simulink model "CrashAlgo_TestEnvironment_Cobi_v1"  (R2020b)
settings: Solver=FixedStepAuto  StartTime=0.0  StopTime=seconds(data.t(end))  FixedStep=0.01  RelTol=1e-3
values from neighbouring files (symbols this model uses):
  CrashClass = <binary blob, 4098 chars, not shown>    [CRCL_Dictionary.sldd]
undefined symbols (not defined in the file or in its folder): data
settings Model: SimulationMode=accelerator  Creator=snj7rt  LastModifiedBy=HNA3SI
settings DebuggingCC: ReadBeforeWriteMsg=DisableAll  WriteAfterWriteMsg=DisableAll  WriteAfterReadMsg=DisableAll  ParameterPrecisionLossMsg=none  ArithmeticOperatorsInVariantConditions=warning
settings ModelReferenceCC: UpdateModelReferenceTargets=IfOutOfDate
settings SFSimCC: SimUseLocalCustomCode=off  CustomCodeUndefinedFunction=UseInterfaceOnly
settings RTWCC: RTWUseLocalCustomCode=off
settings CodeAppCC: StateflowObjectComments=on

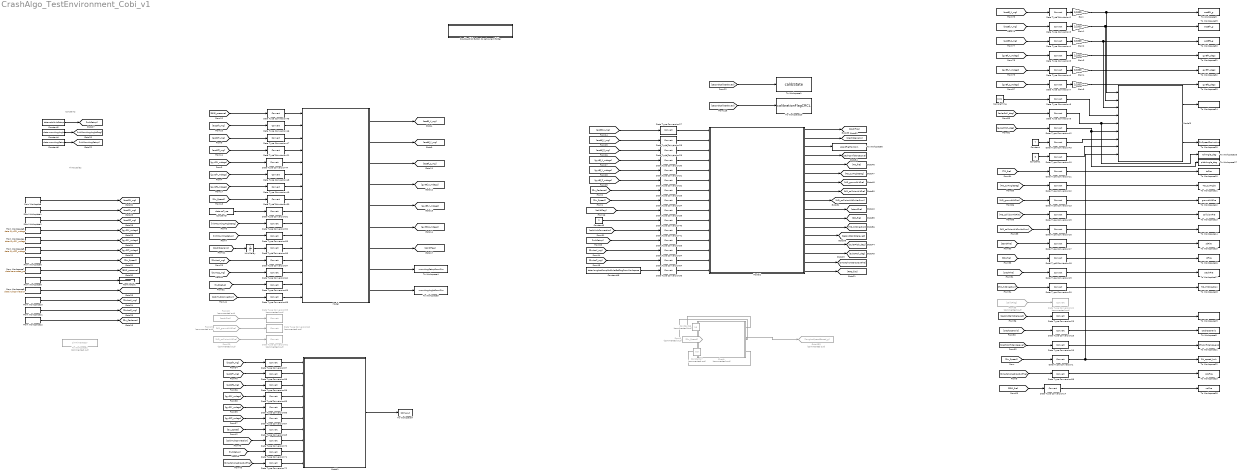
== system CrashAlgo_TestEnvironment_Cobi_v1 ==
  note: Time series
  note: Constants
  Chart1 : Stateflow chart  Commented=on  TreatAsAtomicUnit=on
  Constant : Constant  Value=7
  Constant1 : Constant  Value=5
  Constant2 : Constant  Value=data.cobiHubSetup
  Constant3 : Constant  Value=2
  Constant4 : Constant  Value=data.mountingAngle
  Constant46 : Constant  Commented=on  Value=15
  Constant47 : Constant  Commented=on  Value=0.5
  Constant48 : Constant  Value=data.longAccCompForEulerEstFlagFromWorkspace
  Constant5 : Constant  Value=data.osType
  Constant6 : Constant  Value=data.mountingSetup
  Data Type Conversion{1..20,23,25..26,42..43,58} (26 alike) : DataTypeConversion
  Data Type Conversion{21,27..41,44..57,62..72} (41 alike) : DataTypeConversion  RndMeth=Zero
  Data Type Conversion{22,59..61} (4 alike) : DataTypeConversion  Commented=on
  Double-Click Button to set current folder : Subsystem
      settings: OpenFcn=cd(fileparts(get_param(gcs,'filename')));
      mask Display: disp('\bf\fontsize{16}Double-Click to set current folder      ','texmode','on')
  From Workspace : FromWorkspace  VariableName=data.AccSfX_mg  SampleTime=0.01  Interpolate=off  ZeroCross=off  OutputAfterFinalValue=Setting to zero
  From Workspace1 : FromWorkspace  VariableName=data.AccSfY_mg  SampleTime=0.01  Interpolate=off  ZeroCross=off  OutputAfterFinalValue=Setting to zero
  From Workspace10 : FromWorkspace  VariableName=data.DuAccX_mg  SampleTime=0.01  Interpolate=off  ZeroCross=off  OutputAfterFinalValue=Setting to zero
  From Workspace11 : FromWorkspace  VariableName=data.DuAccZ_mg  SampleTime=0.01  Interpolate=off  ZeroCross=off  OutputAfterFinalValue=Setting to zero
  From Workspace12 : FromWorkspace  VariableName=data.cadence_rpm  SampleTime=0.01  Interpolate=off  ZeroCross=off  OutputAfterFinalValue=Setting to zero
  From Workspace2 : FromWorkspace  VariableName=data.AccSfZ_mg  SampleTime=0.01  Interpolate=off  ZeroCross=off  OutputAfterFinalValue=Setting to zero
  From Workspace3 : FromWorkspace  VariableName=data.GyrSfX_mdegs  SampleTime=0.01  Interpolate=off  ZeroCross=off  OutputAfterFinalValue=Setting to zero
  From Workspace4 : FromWorkspace  VariableName=data.GyrSfY_mdegs  SampleTime=0.01  Interpolate=off  ZeroCross=off  OutputAfterFinalValue=Setting to zero
  From Workspace5 : FromWorkspace  VariableName=data.GyrSfZ_mdegs  SampleTime=0.01  Interpolate=off  ZeroCross=off  OutputAfterFinalValue=Setting to zero
  From Workspace6 : FromWorkspace  VariableName=data.speed_kmh  SampleTime=0.01  Interpolate=off  ZeroCross=off  OutputAfterFinalValue=Setting to zero
  From Workspace7 : FromWorkspace  VariableName=data.barometer_pa  SampleTime=0.01  Interpolate=off  ZeroCross=off  OutputAfterFinalValue=Setting to zero
  From Workspace8 : FromWorkspace  VariableName=data.crashClass  SampleTime=0.01  Interpolate=off  ZeroCross=off  OutputAfterFinalValue=Setting to zero
  From Workspace9 : FromWorkspace  VariableName=data.hubConnection  SampleTime=0.01  Interpolate=off  ZeroCross=off  OutputAfterFinalValue=Setting to zero
  From18 : From  Commented=on  GotoTag=crashFire
  From19 : From  Commented=on  GotoTag=HD_groundHitFire
  From20 : From  Commented=on  GotoTag=HD_collisionHitFire
  From35 : From  Commented=on  GotoTag=calibFlag
  From5 : From  Commented=on  GotoTag=Du_Speed
  Gain{,1..5} (6 alike) : Gain  Gain=1/1000
  Goto153 : Goto  Commented=on  GotoTag=longAccSpeedBased_g
  Model : ModelReference  ModelNameDialog=CobiCalibration.slx  SimulationMode=Normal  ModelReferenceVersion=4.7
  Model1 : ModelReference  ModelNameDialog=SensorDataMonitor.slx  SimulationMode=Normal  ModelReferenceVersion=4.4
  Model2 : ModelReference  ModelNameDialog=CRCL.slx  SimulationMode=Normal  ModelReferenceVersion=4.22
  Model3 : ModelReference  ModelNameDialog=CrashAlgoSchnee_v2_analysis.slx  SimulationMode=Normal  ModelReferenceVersion=4.11
  SampleTime : Constant  Value=0.01
  Terminator1 : Terminator
  To Workspace1 : ToWorkspace  VariableName=calibState  SampleTime=-1
      settings: Save2DSignal=2-D array (concatenate along first dimension)
  To Workspace10 : ToWorkspace  VariableName=toFire  SampleTime=-1
  To Workspace11 : ToWorkspace  VariableName=TO_curAngle  SampleTime=-1
  To Workspace12 : ToWorkspace  VariableName=groundHitFire  SampleTime=-1
  To Workspace13 : ToWorkspace  VariableName=collisionFire  SampleTime=-1
  To Workspace14 : ToWorkspace  VariableName=HD_CollisionCurVarSum  SampleTime=-1
  To Workspace15 : ToWorkspace  VariableName=sdFire  SampleTime=-1
  To Workspace16 : ToWorkspace  VariableName=rdFire  SampleTime=-1
  To Workspace17 : ToWorkspace  VariableName=crashFire  SampleTime=-1
  To Workspace18 : ToWorkspace  VariableName=HD_HitDirection  SampleTime=-1
  To Workspace19 : ToWorkspace  VariableName=SecondCalibrationDelayed  SampleTime=-1
  To Workspace2 : ToWorkspace  Commented=on  VariableName=simTimeVector  SampleTime=-1
      settings: Save2DSignal=2-D array (concatenate along first dimension)
  To Workspace20 : ToWorkspace  VariableName=calibrationFlagCRCL  SampleTime=-1
      settings: Save2DSignal=2-D array (concatenate along first dimension)
  To Workspace21 : ToWorkspace  VariableName=CF_confidenceLevel  SampleTime=-1
  To Workspace22 : ToWorkspace  VariableName=DU_speed_kmh  SampleTime=-1
  To Workspace23 : ToWorkspace  VariableName=sdoFire  SampleTime=-1
  To Workspace24 : ToWorkspace  VariableName=accImpulseXYsquaredSum  SampleTime=-1
  To Workspace25 : ToWorkspace  VariableName=DuSpeedDerivative  SampleTime=-1
  To Workspace26 : ToWorkspace  VariableName=rollAngle_deg  SampleTime=-1
  To Workspace27 : ToWorkspace  VariableName=pitchAngle_deg  SampleTime=-1
  To Workspace28 : ToWorkspace  VariableName=rroFire  SampleTime=-1
  To Workspace29 : ToWorkspace  VariableName=accBfY_g  SampleTime=-1
  To Workspace30 : ToWorkspace  VariableName=accBfZ_g  SampleTime=-1
  To Workspace31 : ToWorkspace  VariableName=gyrBfX_degs  SampleTime=-1
  To Workspace32 : ToWorkspace  VariableName=gyrBfY_degs  SampleTime=-1
  To Workspace33 : ToWorkspace  VariableName=gyrBfZ_degs  SampleTime=-1
  To Workspace4 : ToWorkspace  VariableName=mountingSetupFromSim  SampleTime=-1
      settings: Save2DSignal=2-D array (concatenate along first dimension)
  To Workspace5 : ToWorkspace  VariableName=mountingAngleFromSim  SampleTime=-1
      settings: Save2DSignal=2-D array (concatenate along first dimension)
  To Workspace6 : ToWorkspace  VariableName=abortFireFromSim  SampleTime=-1
      settings: Save2DSignal=2-D array (concatenate along first dimension)
  To Workspace7 : ToWorkspace  VariableName=SDM_out  SampleTime=-1
  To Workspace8 : ToWorkspace  VariableName=crashScenario  SampleTime=-1
  To Workspace9 : ToWorkspace  VariableName=accBfX_g  SampleTime=-1
  Unit Delay : UnitDelay  InitialCondition=CrashClass.crashClassNoCrash  SampleTime=-1  HasFrameUpgradeWarning=on
  wires:
  Data Type Conversion3/1 -> Gain1/1
  [eulerPitch_deg] -> Data Type Conversion42/1
  Data Type Conversion31/1 -> Model2/5
  [standFire] -> Data Type Conversion17/1
  [gyrBf_Y_mdegs] -> Data Type Conversion6/1
  Data Type Conversion29/1 -> Model2/3
  Model2/6 -> [TO_curAngleDeg]  "tipOverAngle_deg"
  Data Type Conversion5/1 -> Gain3/1
  [gyrBf_X_mdegs] -> Data Type Conversion5/1
  [secondCalibDelayed] -> Data Type Conversion23/1
  [gyrBf_Z_mdegs] -> Data Type Conversion7/1
  [HD_collisionHitFire] -> Data Type Conversion15/1
  Data Type Conversion11/1 -> To Workspace10/1
  Data Type Conversion28/1 -> Model2/2
  From35/1 -> Data Type Conversion22/1
  Data Type Conversion7/1 -> Gain5/1
  [HD_groundHitFire] -> Data Type Conversion13/1
  Model2/5 -> [TO_fire]  "TO_fire"
  [crashConfidenceLevel] -> Data Type Conversion26/1
  [Du_Speed] -> Data Type Conversion34/1
  [crashFire] -> Data Type Conversion19/1
  SampleTime/1 -> Data Type Conversion8/1
  Data Type Conversion32/1 -> Model2/6
  Model2/7 -> [HD_groundHitFire]  "HD_GroundHitFire"
  Data Type Conversion43/1 -> Model3/7
  Data Type Conversion34/1 -> Model2/8
  Data Type Conversion27/1 -> Model2/1
  [RD_fire] -> Data Type Conversion18/1
  Data Type Conversion30/1 -> Model2/4
  [Du_Cadence] -> Data Type Conversion33/1
  Data Type Conversion10/1 -> Model3/8
  Data Type Conversion6/1 -> Gain4/1
  [TO_curAngleDeg] -> Data Type Conversion12/1
  [HD_collisionHitCurVarSum] -> Data Type Conversion16/1
  [TO_fire] -> Data Type Conversion11/1
  [accBf_Z_mg] -> Data Type Conversion4/1
  Data Type Conversion2/1 -> Gain/1
  [accBf_X_mg] -> Data Type Conversion2/1
  Model2/4 -> [crashConfidenceLevel]  "crashConfidenceLevel"
  Model2/1 -> [crashFire]  "CrashFire"
  Data Type Conversion13/1 -> To Workspace12/1
  Data Type Conversion35/1 -> Model2/9
  [eulerRoll_deg] -> Data Type Conversion9/1
  Data Type Conversion4/1 -> Gain2/1
  [accBf_Y_mg] -> Data Type Conversion3/1
  [calibFlag] -> Data Type Conversion35/1
  [HD_hitDirection] -> Data Type Conversion20/1
  Data Type Conversion33/1 -> Model2/7
  Data Type Conversion12/1 -> To Workspace11/1
  [Du_Speed] -> Data Type Conversion1/1
  [BMP_pressure] -> Data Type Conversion45/1
  Data Type Conversion45/1 -> Model/1
  Data Type Conversion46/1 -> Model/2
  Data Type Conversion47/1 -> Model/3
  Data Type Conversion21/1 -> Model/4
  Data Type Conversion44/1 -> Model/5
  Data Type Conversion48/1 -> Model/6
  Data Type Conversion49/1 -> Model/7
  Data Type Conversion50/1 -> Model/8
  [gyrSfX_mdegs] -> Data Type Conversion44/1
  [gyrSfY_mdegs] -> Data Type Conversion48/1
  [gyrSfZ_mdegs] -> Data Type Conversion49/1
  Model/1 -> [accBf_X_mg]  "accBfX_mg"
  Model/2 -> [accBf_Y_mg]  "accBfY_mg"
  Model/3 -> [accBf_Z_mg]  "accBfZ_mg"
  Model/4 -> [gyrBf_X_mdegs]  "gyrBfX_mdegs"
  Model/5 -> [gyrBf_Y_mdegs]  "gyrBfY_mdegs"
  Model/6 -> [gyrBf_Z_mdegs]  "gyrBfZ_mdegs"
  Model/7 -> [calibFlag]  "calibFlag"
  [Du_Speed] -> Data Type Conversion50/1
  [accBf_X_mg] -> Data Type Conversion27/1
  [accBf_Y_mg] -> Data Type Conversion28/1
  [accBf_Z_mg] -> Data Type Conversion29/1
  [gyrBf_X_mdegs] -> Data Type Conversion30/1
  [gyrBf_Y_mdegs] -> Data Type Conversion31/1
  [gyrBf_Z_mdegs] -> Data Type Conversion32/1
  [accSfY_mg] -> Data Type Conversion47/1
  [accSfX_mg] -> Data Type Conversion46/1
  [accSfZ_mg] -> Data Type Conversion21/1
  Constant5/1 -> Data Type Conversion51/1
  Data Type Conversion51/1 -> Model/9
  Data Type Conversion52/1 -> Model/10
  Data Type Conversion55/1 -> Model/11
  [initMountingSetup] -> Data Type Conversion55/1
  [SmartphoneDropOutFire] -> Data Type Conversion58/1
  [secondCalibDelayed] -> To Workspace20/1
  From19/1 -> Data Type Conversion60/1
  From18/1 -> Data Type Conversion59/1
  From20/1 -> Data Type Conversion61/1
  [crashScenario] -> Unit Delay/1  "csExtern"
  Data Type Conversion56/1 -> Model/12  "csExtern3"
  Unit Delay/1 -> Data Type Conversion56/1  "csExtern2"
  Model2/2 -> [crashScenario]  "CP_scenario"
  [crashScenario] -> Data Type Conversion25/1
  [secondCalibDelayed] -> To Workspace1/1
  [DuAccX_mg] -> Data Type Conversion57/1
  [DuAccZ_mg] -> Data Type Conversion62/1
  Data Type Conversion57/1 -> Model/13
  Data Type Conversion62/1 -> Model/14
  Data Type Conversion63/1 -> Model/15
  [hubSetup] -> Data Type Conversion63/1
  Model2/3 -> To Workspace6/1  "crashAborted"
  [initMountingAngleDeg] -> Data Type Conversion52/1
  Gain/1 -> Model3/1, To Workspace9/1
  Gain1/1 -> Model3/2, To Workspace29/1
  Gain2/1 -> Model3/3, To Workspace30/1
  Constant3/1 -> Data Type Conversion40/1
  Data Type Conversion40/1 -> Model2/10
  [hubSetup] -> Data Type Conversion53/1
  Data Type Conversion41/1 -> Model2/11
  Data Type Conversion64/1 -> Model2/14
  Data Type Conversion54/1 -> Model2/13
  [DuAccX_mg] -> Data Type Conversion54/1
  Data Type Conversion53/1 -> Model2/12
  [DuAccZ_mg] -> Data Type Conversion64/1
  [cobiHubConnection] -> Data Type Conversion41/1
  Model/8 -> To Workspace4/1  "mountingSetup"
  Model/9 -> To Workspace5/1  "mountingAngle"
  Constant/1 -> Data Type Conversion43/1
  Constant1/1 -> Data Type Conversion10/1
  Model2/8 -> [HD_collisionHitFire]  "HD_CollisionHitFire"
  Model2/9 -> [HD_collisionHitCurVarSum]  "HD_collisionHitCurVarSum"
  Model2/10 -> [standFire]  "SD_StandFire"
  Model2/11 -> [RD_fire]  "RD_fire"
  Model2/12 -> [HD_hitDirection]  "HD_hitDirection"
  Model2/13 -> [secondCalibDelayed]  "secCalibrationDone Delayed"
  Model2/14 -> [eulerPitch_deg]  "eulerPitch_deg"
  Model2/15 -> [eulerRoll_deg]  "eulerRoll_deg"
  Model2/16 -> [SmartphoneDropOutFire]  "SDO_fire"
  From5/1 -> Chart1/2(LAE_curSpeed_kmh)
  Chart1/1(LAE_longAcc_g) -> Goto153/1  "LAE_longAcc_g"
  Constant47/1 -> Chart1/3(LAE_minSpeedDelta_kmh)
  Constant46/1 -> Chart1/1(LAE_minSpeed_kmh)
  Constant48/1 -> Data Type Conversion36/1
  Data Type Conversion36/1 -> Model2/15
  [accSfX_mg] -> Data Type Conversion37/1
  [accSfY_mg] -> Data Type Conversion38/1
  [accSfZ_mg] -> Data Type Conversion39/1
  [gyrSfX_mdegs] -> Data Type Conversion65/1
  [gyrSfY_mdegs] -> Data Type Conversion66/1
  [gyrSfZ_mdegs] -> Data Type Conversion67/1
  Model1/1 -> To Workspace7/1
  Data Type Conversion37/1 -> Model1/1
  Data Type Conversion38/1 -> Model1/2
  Data Type Conversion39/1 -> Model1/3
  Data Type Conversion65/1 -> Model1/4
  Data Type Conversion66/1 -> Model1/5
  Data Type Conversion67/1 -> Model1/6
  Data Type Conversion68/1 -> Model/16
  [cobiHubConnection] -> Data Type Conversion68/1
  [Du_Speed] -> Data Type Conversion69/1
  Data Type Conversion69/1 -> Model1/7
  Data Type Conversion71/1 -> Model1/9
  Data Type Conversion70/1 -> Model1/8
  [hubSetup] -> Data Type Conversion71/1
  [cobiHubConnection] -> Data Type Conversion70/1
  [SmartphoneDropOutFire] -> Data Type Conversion72/1
  Data Type Conversion72/1 -> Model1/10
  Data Type Conversion25/1 -> To Workspace8/1
  Data Type Conversion26/1 -> To Workspace21/1
  Data Type Conversion1/1 -> To Workspace22/1, Model3/9
  Data Type Conversion58/1 -> To Workspace23/1
  Data Type Conversion15/1 -> To Workspace13/1
  Data Type Conversion16/1 -> To Workspace14/1
  Data Type Conversion17/1 -> To Workspace15/1
  Data Type Conversion18/1 -> To Workspace16/1
  Data Type Conversion19/1 -> To Workspace17/1
  Data Type Conversion20/1 -> To Workspace18/1
  Data Type Conversion23/1 -> To Workspace19/1
  Data Type Conversion8/1 -> Model3/4
  Data Type Conversion9/1 -> To Workspace26/1, Model3/5
  Data Type Conversion42/1 -> Model3/6, To Workspace27/1
  Gain3/1 -> To Workspace31/1
  Gain4/1 -> To Workspace32/1
  Gain5/1 -> To Workspace33/1
  Model3/1 -> To Workspace24/1
  Model3/2 -> To Workspace25/1
  Model2/17 -> [RRO_fire]  "RRO_fire"
  Data Type Conversion14/1 -> To Workspace28/1
  [RRO_fire] -> Data Type Conversion14/1
  From Workspace7/1 -> [BMP_pressure]  "BME_pressure"
  From Workspace8/1 -> Terminator1/1  "savedCrashClass"
  From Workspace3/1 -> [gyrSfX_mdegs]  "gyrSfX_mg"
  From Workspace6/1 -> [Du_Speed]  "DuSpeed_kmh"
  From Workspace/1 -> [accSfX_mg]  "accSfXEnv_mg"
  From Workspace1/1 -> [accSfY_mg]  "accSfYEnv_mg"
  From Workspace5/1 -> [gyrSfZ_mdegs]  "gyrSfZ_mg"
  From Workspace2/1 -> [accSfZ_mg]  "accSfZEnv_mg"
  From Workspace4/1 -> [gyrSfY_mdegs]  "gyrSfY_mg"
  Constant2/1 -> [hubSetup]
  From Workspace9/1 -> [cobiHubConnection]  "hubConnection"
  Constant4/1 -> [initMountingAngleDeg]
  Constant6/1 -> [initMountingSetup]
  From Workspace10/1 -> [DuAccX_mg]  "DuAccX_mg"
  From Workspace11/1 -> [DuAccZ_mg]  "DuAccZ_mg"
  From Workspace12/1 -> [Du_Cadence]  "cadence_rpm"

== system CrashAlgo_TestEnvironment_Cobi_v1/Double-Click Button to set current folder ==

== stateflow chart CrashAlgo_TestEnvironment_Cobi_v1/Chart1 ==
  state speedChange
    en:
    LAE_longAcc_g = (LAE_curSpeed_kmh-LAE_lastSpeed_kmh)/(3.6*9.81);
    LAE_lastSpeed_kmh = LAE_curSpeed_kmh;
  state Idle
    du:
    LAE_lastSpeed_kmh = LAE_curSpeed_kmh;
  (default) -> Idle : {
      | LAE_lastSpeed_kmh = single(0);
      | LAE_longAcc_g = single(0);
      | }
  Idle -> speedChange [order 1] : %decelerating
      | [LAE_lastSpeed_kmh-LAE_curSpeed_kmh > LAE_minSpeedDelta_kmh && ...
      | (LAE_curSpeed_kmh >= LAE_minSpeed_kmh || ...
      |  LAE_lastSpeed_kmh >= LAE_minSpeed_kmh)]
  Idle -> speedChange [order 2] : %accelerating
      | [LAE_curSpeed_kmh-LAE_lastSpeed_kmh > LAE_minSpeedDelta_kmh && ...
      |  LAE_lastSpeed_kmh >= LAE_minSpeed_kmh]
  speedChange -> Idle
  Idle -> Idle [order 3] : [after(1,sec)]
      | {
      | LAE_longAcc_g = single(0);
      | }
  data: LAE_minSpeed_kmh input; LAE_curSpeed_kmh input; LAE_minSpeedDelta_kmh input; LAE_longAcc_g output; LAE_lastSpeed_kmh local
